simulink model "Controlador_Movimiento_PID"  (R2023b)
settings: Solver=VariableStepAuto  StartTime=0.0  StopTime=10.0  RelTol=1e-3
undefined symbols (not defined in the file or in its folder): k_d, K_i, K_p
settings Model: Creator=ignab  LastModifiedBy=ignab

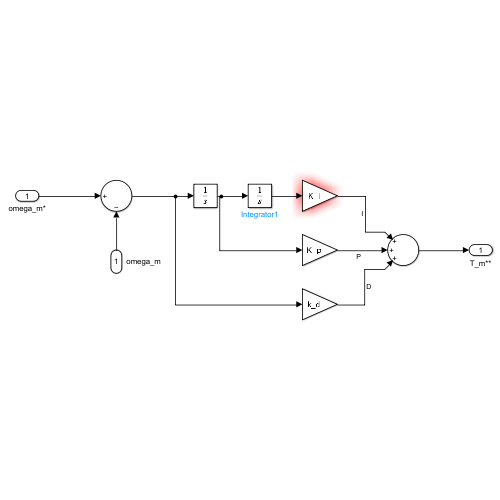
[thumbnail: Simulink's stored preview of the top-level diagram]
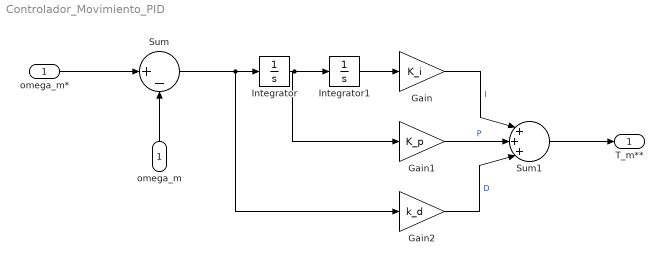
== system Controlador_Movimiento_PID ==
  omega_m* : Inport
  Gain : Gain  Gain=K_i
  Gain1 : Gain  Gain=K_p
  Gain2 : Gain  Gain=k_d
  Integrator : Integrator
  Integrator1 : Integrator
  Sum : Sum  Inputs=|+-
  Sum1 : Sum  Inputs=|+++|
  omega_m : InportShadow
  T_m** : Outport
  wires:
  Sum/1 -> Gain2/1, Integrator/1
  omega_m/1 -> Sum/2
  omega_m*/1 -> Sum/1
  Integrator/1 -> Gain1/1, Integrator1/1
  Integrator1/1 -> Gain/1
  Sum1/1 -> T_m**/1
  Gain/1 -> Sum1/1  "I"
  Gain1/1 -> Sum1/2  "P"
  Gain2/1 -> Sum1/3  "D"
